simulink model "GalvoModel_v3_discret_simo_GUT_ohne_satt"  (R2013a)
settings: Solver=ode45  StartTime=0.0  StopTime=20e-3  MaxStep=1e-6  RelTol=1e-3
values from neighbouring files (symbols this model uses):
  BEM = 108e-6    (= 0.000108)    [GalvoModel_WOK_step.m]
  CL = 180e-6    (= 0.00018)    [GalvoModel_WOK_step.m]    (also in GalvoModel_v4_sys.m = @(x,n) repmat(x, 1, n); GalvoModel_v6_sys.m = @(x,n) repmat(x, 1, n))
  CR = 2.79    [GalvoModel_WOK_step.m]
  FR = 4e-12    [GalvoModel_WOK_step.m]
  KTR = 47e-3    (= 0.047)    [GalvoModel_WOK_step.m]
  RIN = 1.25e-8    (= 1.25e-08)    [GalvoModel_WOK_step.m]
  TRC = 6.17e-3    (= 0.00617)    [GalvoModel_WOK_step.m]
libraries: simulink x2
settings Model: Creator=mainster  LastModifiedBy=mainster
settings DebuggingCC: SolverPrmCheckMsg=none

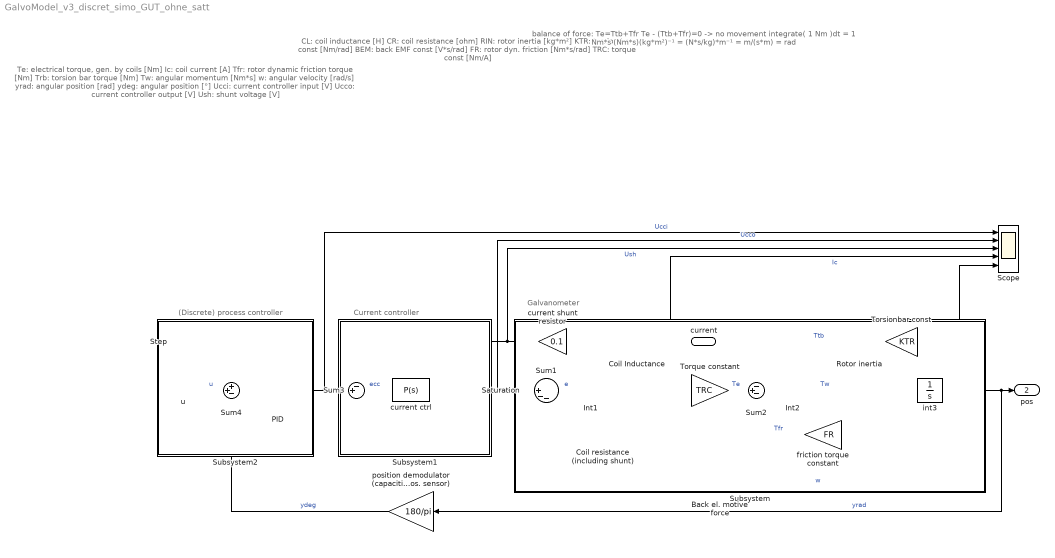
== system GalvoModel_v3_discret_simo_GUT_ohne_satt ==
  note: Current controller
  note: Galvanometer
  note: Te: 		electrical torque, gen. by coils		[Nm]
      |  Ic: 			coil current							[A]
      |  Tfr:		rotor dynamic friction torque 		[Nm]
      |  Trb:		torsion bar torque					[Nm]
      |  Tw:		angular momentum				[Nm*s]
      |  w:			angular velocity 					[rad/s]
      |  yrad:		angular position 					[rad]
      |  ydeg:		angular position 					[°]
      |  Ucci:		current controller input				[V]
      |  Ucco:		current controller output			[V]
      |  Ush:		shunt voltage						[V]
  note: CL:	coil inductance 		[H]
      |  CR:	coil resistance 			[ohm]
      |  RIN:	rotor inertia 			[kg*m²]
      |  KTR:	torsion bar const 		[Nm/rad]
      |  BEM:	back EMF const		[V*s/rad]
      |  FR:	rotor dyn. friction		[Nm*s/rad]
      |  TRC:	torque const			[Nm/A]
  note: balance of force: 	Te=Ttb+Tfr
      | 					Te - (Ttb+Tfr)=0  ->  no movement
      |
      |  integrate( 1 Nm )dt = 1 Nm*s
      |  (Nm*s)(kg*m²)⁻¹ = (N*s/kg)*m⁻¹ = m/(s*m) = rad
  note: (Discrete) process controller
  u : Inport
  Back el. motive force : Gain  Gain=BEM
  Coil Inductance : Gain  Gain=1/CL
  Coil resistance (including shunt) : Gain  Gain=CR
  Int1 : Integrator
  Int2 : Integrator
  PID : simulink/Continuous/PID Controller  Controller=PID  TimeDomain=Continuous-time  SampleTime=1  IntegratorMethod=Forward Euler  FilterMethod=Forward Euler  Form=Parallel  P=0.118803398901385  I=41.4515194383798  D=8.41592067923308e-05  N=758717.459878032  InitialConditionSource=internal  InitialConditionForIntegrator=0  InitialConditionForFilter=0  ExternalReset=none  LimitOutput=on  UpperSaturationLimit=10  LowerSaturationLimit=-10  LinearizeAsGain=off  AntiWindupMode=none  Kb=1  TrackingMode=off  Kt=0  PParamMin=[]  PParamMax=[]  IParamMin=[]  IParamMax=[]  DParamMin=[]  DParamMax=[]  NParamMin=[]  NParamMax=[]  KbParamMin=[]  KbParamMax=[]  KtParamMin=[]  KtParamMax=[]  POutMin=[]  POutMax=[]  IOutMin=[]  IOutMax=[]  DOutMin=[]  DOutMax=[]  NOutMin=[]  NOutMax=[]  KbOutMin=[]  KbOutMax=[]  KtOutMin=[]  KtOutMax=[]  IntegratorOutMin=[]  IntegratorOutMax=[]  FilterOutMin=[]  FilterOutMax=[]  SumOutMin=[]  SumOutMax=[]  SumI1OutMin=[]  SumI1OutMax=[]  SumI2OutMin=[]  SumI2OutMax=[]  SumI3OutMin=[]  SumI3OutMax=[]  SumDOutMin=[]  SumDOutMax=[]  SaturationOutMin=[]  SaturationOutMax=[]  IntegratorContinuousStateAttributes=''  IntegratorStateMustResolveToSignalObject=off  IntegratorRTWStateStorageClass=Auto  FilterContinuousStateAttributes=''  FilterStateMustResolveToSignalObject=off  FilterRTWStateStorageClass=Auto
  Rotor inertia : Gain  Gain=1/RIN
  Saturation : Saturate  UpperLimit=25e9  LowerLimit=-25e9
      settings: AttributesFormatString=Saturation:\n<%<LowerLimit>\n>%<UpperLimit>
  Scope : Scope  NumInputPorts=5
      settings: ShowLegends=on  TimeRange=0.02  YMin=-5~-5~-5~-5~-5  YMax=5~5~5~5~5  MaxDataPoints=500000
  Step : Step  Time=1e-3  After=2  SampleTime=0
      settings: AttributesFormatString=Ampl.: %<After>
  Subsystem : Subsystem  mask{d=0}
      mask Display: disp('')
  Subsystem1 : Subsystem  mask{d=0}
      mask Display: disp('')
  Subsystem2 : Subsystem  mask{d=0}
      mask Display: disp('')
  Sum1 : Sum  Inputs=||+--
  Sum2 : Sum  Inputs=-+-
  Sum3 : Sum  Inputs=-+|
  Sum4 : Sum  Inputs=++-
  Torque constant : Gain  Gain=TRC
  Torsionbar const : Gain  Gain=KTR
  current ctrl : simulink/Continuous/PID Controller  Controller=P  TimeDomain=Continuous-time  SampleTime=1  IntegratorMethod=Forward Euler  FilterMethod=Forward Euler  Form=Parallel  P=10  I=0.7525  D=0.156  N=100  InitialConditionSource=internal  InitialConditionForIntegrator=0  InitialConditionForFilter=0  ExternalReset=none  LimitOutput=on  UpperSaturationLimit=25  LowerSaturationLimit=-25  LinearizeAsGain=off  AntiWindupMode=none  Kb=1  TrackingMode=off  Kt=1  PParamMin=[]  PParamMax=[]  IParamMin=[]  IParamMax=[]  DParamMin=[]  DParamMax=[]  NParamMin=[]  NParamMax=[]  KbParamMin=[]  KbParamMax=[]  KtParamMin=[]  KtParamMax=[]  POutMin=[]  POutMax=[]  IOutMin=[]  IOutMax=[]  DOutMin=[]  DOutMax=[]  NOutMin=[]  NOutMax=[]  KbOutMin=[]  KbOutMax=[]  KtOutMin=[]  KtOutMax=[]  IntegratorOutMin=[]  IntegratorOutMax=[]  FilterOutMin=[]  FilterOutMax=[]  SumOutMin=[]  SumOutMax=[]  SumI1OutMin=[]  SumI1OutMax=[]  SumI2OutMin=[]  SumI2OutMax=[]  SumI3OutMin=[]  SumI3OutMax=[]  SumDOutMin=[]  SumDOutMax=[]  SaturationOutMin=[]  SaturationOutMax=[]  IntegratorContinuousStateAttributes=''  IntegratorStateMustResolveToSignalObject=off  IntegratorRTWStateStorageClass=Auto  FilterContinuousStateAttributes=''  FilterStateMustResolveToSignalObject=off  FilterRTWStateStorageClass=Auto
  current shunt resistor : Gain  Gain=0.1
  friction torque constant : Gain  Gain=FR
  int3 : Integrator
  position demodulator (capacitive angular pos. sensor) : Gain  Gain=180/pi
  current : Outport
  pos : Outport  Port=2
  wires:
  int3/1 -> Scope/5, Torsionbar const/1, pos/1, position demodulator (capacitive angular pos. sensor)/1  "yrad"
  Torque constant/1 -> Sum2/2  "Te"
  Sum3/1 -> current ctrl/1  "ecc"
  current shunt resistor/1 -> Scope/3, Sum3/1  "Ush"
  PID/1 -> Scope/1, Sum3/2  "Ucci"
  Sum4/1 -> PID/1
  Coil Inductance/1 -> Scope/4, current shunt resistor/1, current/1, Torque constant/1, Coil resistance (including shunt)/1  "Ic"
  Torsionbar const/1 -> Sum2/1  "Ttb"
  current ctrl/1 -> Saturation/1
  Step/1 -> Sum4/1
  u/1 -> Sum4/2  "u"
  position demodulator (capacitive angular pos. sensor)/1 -> Sum4/3  "ydeg"
  Int1/1 -> Coil Inductance/1
  Coil resistance (including shunt)/1 -> Sum1/3
  Sum1/1 -> Int1/1  "e"
  Int2/1 -> Rotor inertia/1  "Tw"
  Sum2/1 -> Int2/1
  Rotor inertia/1 -> int3/1, Back el. motive force/1, friction torque constant/1  "w"
  friction torque constant/1 -> Sum2/3  "Tfr"
  Back el. motive force/1 -> Sum1/2
  Saturation/1 -> Scope/2, Sum1/1  "Ucco"

== system GalvoModel_v3_discret_simo_GUT_ohne_satt/Subsystem ==

== system GalvoModel_v3_discret_simo_GUT_ohne_satt/Subsystem1 ==

== system GalvoModel_v3_discret_simo_GUT_ohne_satt/Subsystem2 ==
